simulink model "Eco_sensor"  (R2018a)
settings: Solver=VariableStepAuto  StartTime=0.0  StopTime=10.0  RelTol=1e-3
PreLoadFcn:
  | % Create Parameters
  | degConv = 180/pi;
  | t = linspace(0,10,101)';
  | u = linspace(0,pi/2,101)';
settings Model: Creator=Tom  LastModifiedBy=Tom
settings DataIOCC: LoadExternalInput=on

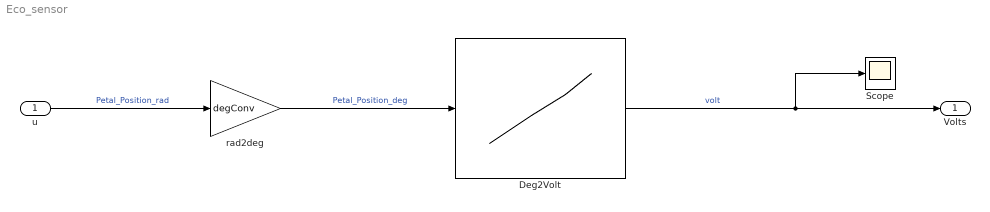
== system Eco_sensor ==
  u : Inport
  Deg2Volt : Lookup_n-D  NumberOfTableDimensions=1  BreakpointsForDimension1=[0 90]  Table=[0.5 4.5]  ExtrapMethod=Clip  InternalRulePriority=Speed  RndMeth=Simplest  InputSameDT=on
  Scope : Scope
  rad2deg : Gain  Gain=degConv
  Volts : Outport
  wires:
  u/1 -> rad2deg/1  "Petal_Position_rad"
  rad2deg/1 -> Deg2Volt/1  "Petal_Position_deg"
  Deg2Volt/1 -> Volts/1, Scope/1  "volt"
